simulink model "r"  (R2013a)
settings: Solver=ode23tb  StartTime=0.0  StopTime=2/60  RelTol=1e-3
values from neighbouring files (symbols this model uses):
  alfa = x(i)    [sim2.m]    (also in sim2rc.m = 60; sim2rl.m = 60)
  R = 50    [sim2.m]    (also in sim2rc.m; sim2rl.m)
  V_source = 100    [sim2.m]    (also in sim2rc.m; sim2rl.m)
libraries: powerlib x8, powerlib_meascontrol x6
settings Model: Creator=dello  LastModifiedBy=dello
settings DataIOCC: SignalLoggingSaveFormat=ModelDataLogs  SignalLoggingName=monofasico
settings OptimizationCC: BlockReduction=off

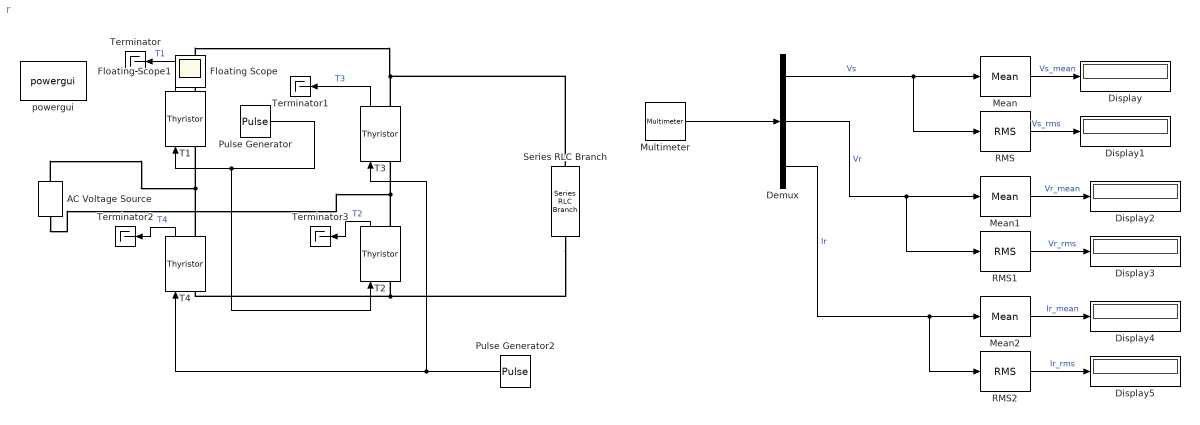
== system r ==
  AC Voltage Source : powerlib/Electrical Sources/AC Voltage Source  Amplitude=V_source  Phase=0  Frequency=60  SampleTime=0  Measurements=Voltage
  Demux : Demux  Outputs=3
  Display{,1..5} (6 alike) : Display
  Mean : powerlib_meascontrol/Measurements/Mean  Freq=60  Vinit=0  Ts=0
  Mean1 : powerlib_meascontrol/Measurements/Mean  Freq=60  Vinit=0  Ts=0
  Mean2 : powerlib_meascontrol/Measurements/Mean  Freq=60  Vinit=0  Ts=0
  Multimeter : powerlib/Measurements/Multimeter  PhasorSimulation=off  OutputType=Complex  sel=[2 1 3]  L=3  Gain=[1 1 1]  yselected={'Usrc: AC Voltage Source','Ub: Series RLC Branch','Ib: Series RLC Branch'};  PSBOutputType=1  PSBequivalent=0  AxesSetting=[0,0.1,-100,100]  Display=0  SavedBlockNames=-11
  Pulse Generator : DiscretePulseGenerator  PulseType=Time based  Period=1/60  PulseWidth=5  PhaseDelay=alfa/360/60
  Pulse Generator2 : DiscretePulseGenerator  PulseType=Time based  Period=1/60  PulseWidth=5  PhaseDelay=(alfa + 180)/360/60
  RMS : powerlib_meascontrol/Measurements/RMS  TrueRMS=on  Freq=60  RMSInit=120  Ts=0
  RMS1 : powerlib_meascontrol/Measurements/RMS  TrueRMS=on  Freq=60  RMSInit=120  Ts=0
  RMS2 : powerlib_meascontrol/Measurements/RMS  TrueRMS=on  Freq=60  RMSInit=120  Ts=0
  Series RLC Branch : powerlib/Elements/Series RLC Branch  LConnTagsString=__new0  RConnTagsString=__new0  BranchType=R  Resistance=R  Inductance=1e-3  SetiL0=off  InitialCurrent=0  Capacitance=1e-6  Setx0=off  InitialVoltage=0  Measurements=Branch voltage and current
  T{1..4} (4 alike) : powerlib/Power Electronics/Thyristor  Ron=0.001  Lon=0  Vf=0.8  IC=0  Rs=500  Cs=250e-9  Measurements=on
  Terminator{,1..3} (4 alike) : Terminator
  powergui : powerlib/powergui  Priority=1  SimulationMode=Continuous  SolverType=Tustin  SampleTime=50e-6  frequency=60  SPID=off  DisableSnubberDevices=off  DisableRonSwitches=off  DisableVfSwitches=off  SwTol=0  Interpol=off  DisplayEquations=off  frequencyindice=60  Pbase=100e6  ErrMax=1e-4  Iterations=50  UnitsV=V  UnitsW=W  FunctionMessages=off  echomessages=off  HookPort=off  EnableUseOfTLC=off  x0status=blocks  RestoreLinks=warning  ResistiveCurrentMeasurement=off  Frange=[0:2:500]  Ylog=off  Xlog=on  ShowGrid=off  save=off  variable=ZData  ZoomFFT=off  StartTime=0.0  cycles=1  DisplayStyle=1  fundamental=60  FreqAxis=off  MaxFrequency=1000  frequencyindicesteady=1  RmsSteady=1  display=off  Ts=0  methode=off
  Floating Scope : Scope  NumInputPorts=8
      settings: Floating=on  TimeRange=0.03333333333333333  YMin=-5~-5~-5~-5~-5~-5~-5~-5  YMax=5~5~5~5~5~5~5~5  SaveName=diodes
  Floating Scope1 : Scope
      settings: Floating=on  TimeRange=0.03333333333333333  SaveName=simdata
  wires:
  Multimeter/1 -> Demux/1
  Demux/1 -> RMS/1, Mean/1  "Vs"
  Demux/2 -> RMS1/1, Mean1/1  "Vr"
  Demux/3 -> RMS2/1, Mean2/1  "Ir"
  Mean/1 -> Display/1  "Vs_mean"
  RMS/1 -> Display1/1  "Vs_rms"
  Mean1/1 -> Display2/1  "Vr_mean"
  RMS1/1 -> Display3/1  "Vr_rms"
  Mean2/1 -> Display4/1  "Ir_mean"
  RMS2/1 -> Display5/1  "Ir_rms"
  T1/1 -> Terminator/1  "T1"
  T3/1 -> Terminator1/1  "T3"
  T2/1 -> Terminator3/1  "T2"
  T4/1 -> Terminator2/1  "T4"
  Pulse Generator/1 -> T2/1, T1/1
  Pulse Generator2/1 -> T3/1, T4/1
  connections:
  AC Voltage Source/RConn1 -- T4/RConn1 -- T1/LConn1
  AC Voltage Source/LConn1 -- T2/RConn1 -- T3/LConn1
  Series RLC Branch/LConn1 -- T3/RConn1 -- T1/RConn1
  Series RLC Branch/RConn1 -- T4/LConn1 -- T2/LConn1
